simulink model "lab3excercise1"  (R2022a)
settings: Solver=VariableStepAuto  StartTime=0.0  StopTime=10.0  RelTol=1e-3
InitFcn:
  | a = Jeq + m*r^2 + ng*(Kg^2)*Jm;
  | b = m*L*r;
  | c = (4/3)m(L^2);
  | d = m*g*L;
  | f = (nm*ng*Kt*Kg)/R;
  | 
  | Jeq = 1.84e-6;
  | m = 0.0270;
  | r = 0.0826;
  | Kg = 1;
  | Jm = 1.80e-4;
  | ng = 1;
  | nm = 0.69;
  | L = 0.0955;
  | g = 9.8;
  | Kt = 0.0344;
  | R = 8.7;
settings Model: Creator=ahmed  LastModifiedBy=ahmed

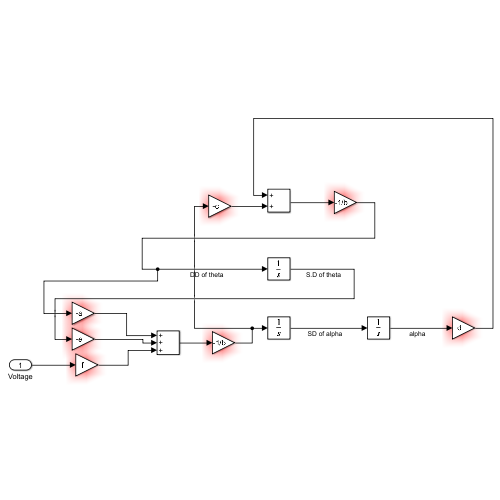
[thumbnail: Simulink's stored preview of the top-level diagram]
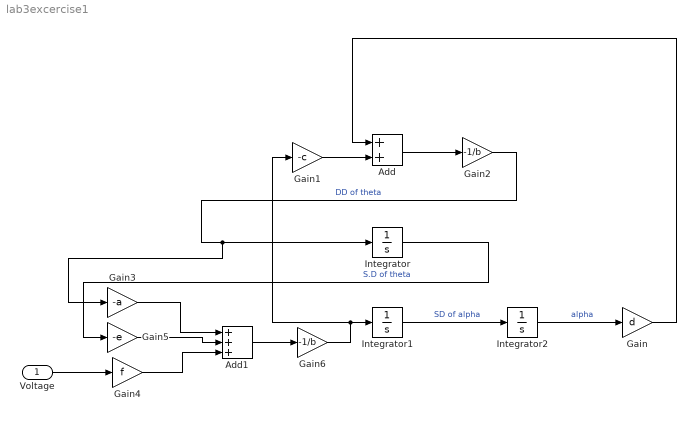
== system lab3excercise1 ==
  Voltage : Inport
  Add : Sum
  Add1 : Sum  Inputs=+++
  Gain : Gain  Gain=d
  Gain1 : Gain  Gain=-c
  Gain2 : Gain  Gain=-1/b
  Gain3 : Gain  Gain=-a
  Gain4 : Gain  Gain=f
  Gain5 : Gain  Gain=-e
  Gain6 : Gain  Gain=-1/b
  Integrator : Integrator
  Integrator1 : Integrator
  Integrator2 : Integrator
  wires:
  Gain2/1 -> Gain3/1, Integrator/1  "DD of theta"
  Integrator/1 -> Gain5/1  "S.D of theta"
  Integrator1/1 -> Integrator2/1  "SD of alpha"
  Integrator2/1 -> Gain/1  "alpha"
  Gain/1 -> Add/1
  Gain1/1 -> Add/2
  Add/1 -> Gain2/1
  Gain4/1 -> Add1/3
  Voltage/1 -> Gain4/1
  Gain5/1 -> Add1/2
  Add1/1 -> Gain6/1
  Gain6/1 -> Integrator1/1, Gain1/1
  Gain3/1 -> Add1/1
